simulink subsystem "rss_PhiSensFaltDiaHybr"  (R2023a)
settings: Solver=VariableStepAuto  StartTime=0.0  StopTime=10.0  RelTol=1e-3
undefined symbols (not defined in the file): ENM_AG_POS_EVAL_MODE, ENM_TYPE_FALT, Gu16_ctPhiSensFaltConfCnt_C, Gu16_ctPhiSensFaltRcvyCnt_C
libraries: simulink x1, lib_debounce x1, lib_fault_definiteness x1
settings Model: Creator=xiaoqiang.yuan  LastModifiedBy=xiaoqiang.yuan

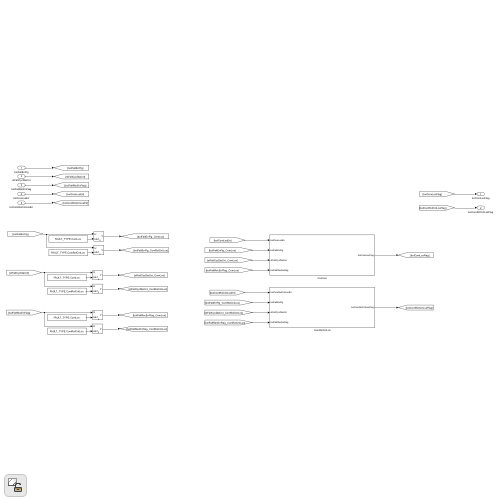
[thumbnail: Simulink's stored preview of the top-level diagram]
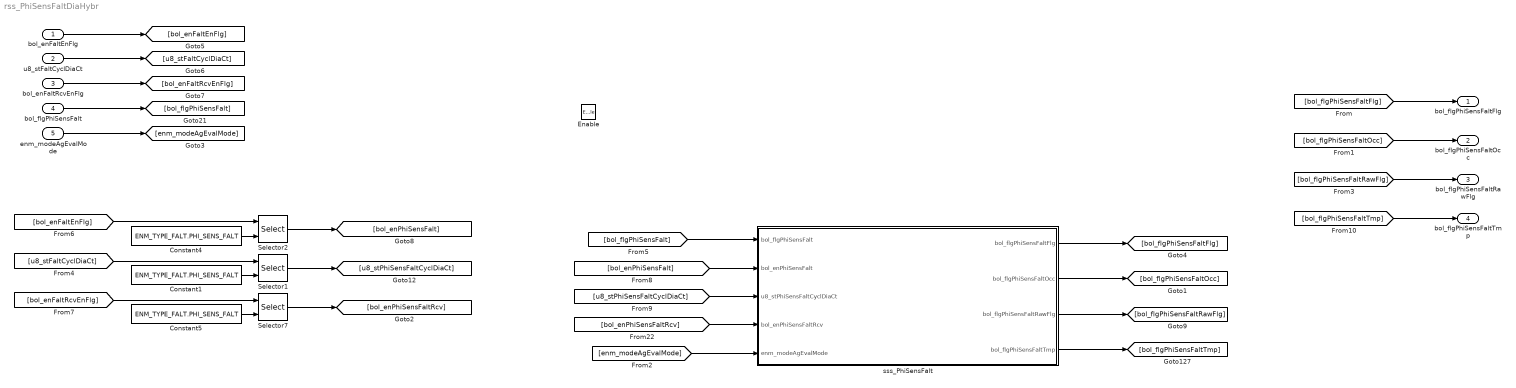
== system rss_PhiSensFaltDiaHybr ==
  bol_enFaltEnFlg : Inport  OutDataTypeStr=boolean
  u8_stFaltCyclDiaCt : Inport  Port=2  OutDataTypeStr=uint8
  bol_enFaltRcvEnFlg : Inport  Port=3  OutDataTypeStr=boolean
  bol_flgPhiSensFalt : Inport  Port=4  OutDataTypeStr=boolean
  enm_modeAgEvalMode : Inport  Port=5  OutDataTypeStr=Enum: ENM_AG_POS_EVAL_MODE
  Enable : EnablePort
  Constant1 : Constant  Value=ENM_TYPE_FALT.PHI_SENS_FALT
  Constant4 : Constant  Value=ENM_TYPE_FALT.PHI_SENS_FALT
  Constant5 : Constant  Value=ENM_TYPE_FALT.PHI_SENS_FALT
  Selector1 : Selector  IndexMode=Zero-based  InputPortWidth=Cdbl_numFaltDiaNum  IndexOptions=Index vector (port)  Indices=[1 3]  OutputSizes=1
  Selector2 : Selector  IndexMode=Zero-based  InputPortWidth=Cdbl_numFaltDiaNum  IndexOptions=Index vector (port)  Indices=[1 3]  OutputSizes=1
  Selector7 : Selector  IndexMode=Zero-based  InputPortWidth=Cdbl_numFaltDiaNum  IndexOptions=Index vector (port)  Indices=[1 3]  OutputSizes=1
  sss_PhiSensFalt : Subsystem
  bol_flgPhiSensFaltFlg : Outport  OutDataTypeStr=boolean
  bol_flgPhiSensFaltOcc : Outport  Port=2  OutDataTypeStr=boolean
  bol_flgPhiSensFaltRawFlg : Outport  Port=3  OutDataTypeStr=boolean
  bol_flgPhiSensFaltTmp : Outport  Port=4  OutDataTypeStr=boolean
  wires:
  [bol_flgPhiSensFaltFlg] -> bol_flgPhiSensFaltFlg/1
  [u8_stFaltCyclDiaCt] -> Selector1/1
  [bol_enFaltEnFlg] -> Selector2/1
  bol_enFaltEnFlg/1 -> [bol_enFaltEnFlg]
  bol_enFaltRcvEnFlg/1 -> [bol_enFaltRcvEnFlg]
  [bol_flgPhiSensFalt] -> sss_PhiSensFalt/1(bol_flgPhiSensFalt)
  Constant1/1 -> Selector1/2
  [u8_stPhiSensFaltCyclDiaCt] -> sss_PhiSensFalt/3(u8_stPhiSensFaltCyclDiaCt)
  [bol_enPhiSensFalt] -> sss_PhiSensFalt/2(bol_enPhiSensFalt)
  Constant4/1 -> Selector2/2
  Constant5/1 -> Selector7/2
  Selector1/1 -> [u8_stPhiSensFaltCyclDiaCt]
  bol_flgPhiSensFalt/1 -> [bol_flgPhiSensFalt]
  Selector7/1 -> [bol_enPhiSensFaltRcv]
  [bol_enFaltRcvEnFlg] -> Selector7/1
  Selector2/1 -> [bol_enPhiSensFalt]
  [bol_enPhiSensFaltRcv] -> sss_PhiSensFalt/4(bol_enPhiSensFaltRcv)
  u8_stFaltCyclDiaCt/1 -> [u8_stFaltCyclDiaCt]
  sss_PhiSensFalt/1(bol_flgPhiSensFaltFlg) -> [bol_flgPhiSensFaltFlg]
  sss_PhiSensFalt/2(bol_flgPhiSensFaltOcc) -> [bol_flgPhiSensFaltOcc]
  [bol_flgPhiSensFaltOcc] -> bol_flgPhiSensFaltOcc/1
  enm_modeAgEvalMode/1 -> [enm_modeAgEvalMode]
  [enm_modeAgEvalMode] -> sss_PhiSensFalt/5(enm_modeAgEvalMode)
  sss_PhiSensFalt/3(bol_flgPhiSensFaltRawFlg) -> [bol_flgPhiSensFaltRawFlg]
  [bol_flgPhiSensFaltRawFlg] -> bol_flgPhiSensFaltRawFlg/1
  [bol_flgPhiSensFaltTmp] -> bol_flgPhiSensFaltTmp/1
  sss_PhiSensFalt/4(bol_flgPhiSensFaltTmp) -> [bol_flgPhiSensFaltTmp]

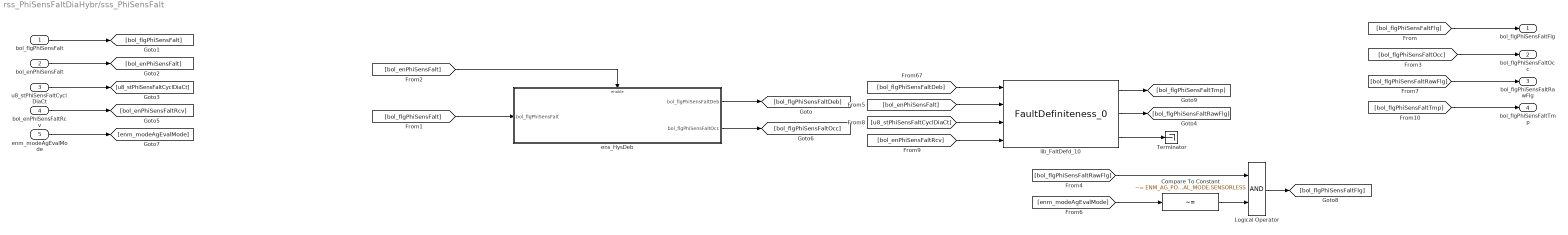
== system rss_PhiSensFaltDiaHybr/sss_PhiSensFalt ==
  bol_flgPhiSensFalt : Inport
  bol_enPhiSensFalt : Inport  Port=2
  u8_stPhiSensFaltCyclDiaCt : Inport  Port=3
  bol_enPhiSensFaltRcv : Inport  Port=4
  enm_modeAgEvalMode : Inport  Port=5
  Compare To Constant : simulink/Logic and Bit Operations/Compare To Constant  relop=~=  const=ENM_AG_POS_EVAL_MODE.SENSORLESS  OutDataTypeStr=boolean
  Logical Operator : Logic  AllPortsSameDT=off  OutDataTypeStr=boolean
  Terminator : Terminator
  ens_HysDeb : Subsystem
  lib_FaltDefd_10 : lib_fault_definiteness/FaultDefiniteness_0  lb_FaltWaitRecvCnt=Gu16_ctPhiSensFaltConfCnt_C
  bol_flgPhiSensFaltFlg : Outport
  bol_flgPhiSensFaltOcc : Outport  Port=2
  bol_flgPhiSensFaltRawFlg : Outport  Port=3
  bol_flgPhiSensFaltTmp : Outport  Port=4
  wires:
  [bol_flgPhiSensFaltTmp] -> bol_flgPhiSensFaltTmp/1
  [bol_flgPhiSensFaltRawFlg] -> bol_flgPhiSensFaltRawFlg/1
  Logical Operator/1 -> [bol_flgPhiSensFaltFlg]
  [bol_flgPhiSensFaltRawFlg] -> Logical Operator/1
  Compare To Constant/1 -> Logical Operator/2
  [enm_modeAgEvalMode] -> Compare To Constant/1
  enm_modeAgEvalMode/1 -> [enm_modeAgEvalMode]
  [bol_flgPhiSensFaltOcc] -> bol_flgPhiSensFaltOcc/1
  ens_HysDeb/2(bol_flgPhiSensFaltOcc) -> [bol_flgPhiSensFaltOcc]
  lib_FaltDefd_10/1 -> [bol_flgPhiSensFaltTmp]
  lib_FaltDefd_10/2 -> [bol_flgPhiSensFaltRawFlg]
  lib_FaltDefd_10/3 -> Terminator/1
  [bol_enPhiSensFalt] -> ens_HysDeb/Enable
  [bol_flgPhiSensFalt] -> ens_HysDeb/1(bol_flgPhiSensFalt)
  ens_HysDeb/1(bol_flgPhiSensFaltDeb) -> [bol_flgPhiSensFaltDeb]
  bol_enPhiSensFaltRcv/1 -> [bol_enPhiSensFaltRcv]
  u8_stPhiSensFaltCyclDiaCt/1 -> [u8_stPhiSensFaltCyclDiaCt]
  bol_enPhiSensFalt/1 -> [bol_enPhiSensFalt]
  [bol_flgPhiSensFaltFlg] -> bol_flgPhiSensFaltFlg/1
  bol_flgPhiSensFalt/1 -> [bol_flgPhiSensFalt]
  [bol_enPhiSensFaltRcv] -> lib_FaltDefd_10/4
  [u8_stPhiSensFaltCyclDiaCt] -> lib_FaltDefd_10/3
  [bol_enPhiSensFalt] -> lib_FaltDefd_10/2
  [bol_flgPhiSensFaltDeb] -> lib_FaltDefd_10/1

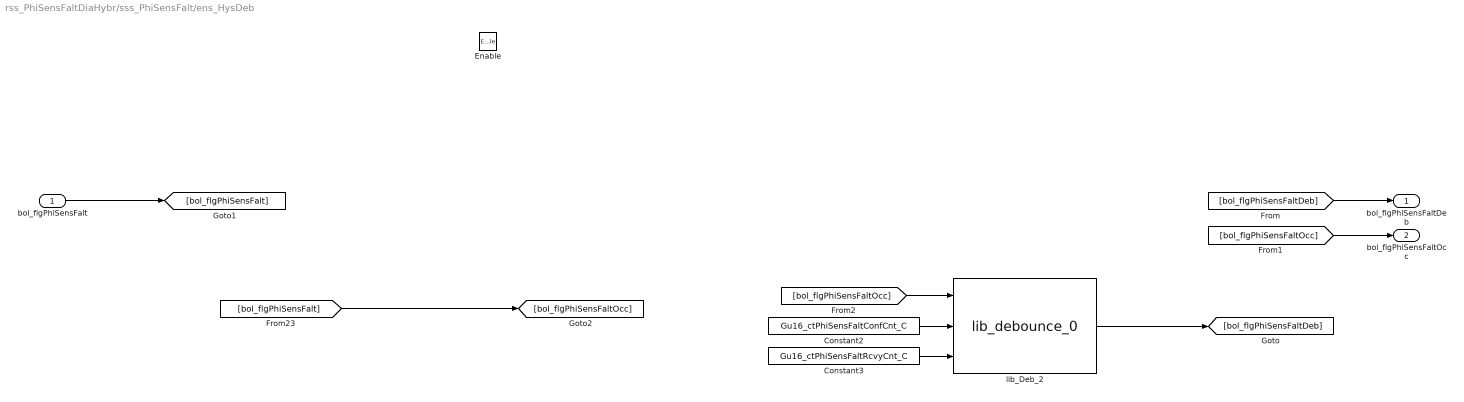
== system rss_PhiSensFaltDiaHybr/sss_PhiSensFalt/ens_HysDeb ==
  bol_flgPhiSensFalt : Inport
  Enable : EnablePort
  Constant2 : Constant  Value=Gu16_ctPhiSensFaltConfCnt_C
  Constant3 : Constant  Value=Gu16_ctPhiSensFaltRcvyCnt_C
  lib_Deb_2 : lib_debounce/lib_debounce_0
  bol_flgPhiSensFaltDeb : Outport
  bol_flgPhiSensFaltOcc : Outport  Port=2
  wires:
  [bol_flgPhiSensFaltOcc] -> lib_Deb_2/1
  [bol_flgPhiSensFalt] -> [bol_flgPhiSensFaltOcc]
  [bol_flgPhiSensFaltOcc] -> bol_flgPhiSensFaltOcc/1
  lib_Deb_2/1 -> [bol_flgPhiSensFaltDeb]
  bol_flgPhiSensFalt/1 -> [bol_flgPhiSensFalt]
  [bol_flgPhiSensFaltDeb] -> bol_flgPhiSensFaltDeb/1
  Constant3/1 -> lib_Deb_2/3
  Constant2/1 -> lib_Deb_2/2
